simulink model "Reverse_Osmosis_2_pass_R2016a"  (R2022b)
settings: Solver=VariableStepAuto  StartTime=0.0  StopTime=7*3600  RelTol=1e-3
model workspace (MAT data in the model file):
  H2_D = 74
  H2_R = 4124.48151676
  H2_T = [-56.55 -50 -40 -30 -20 -10 -5 -4 -3 -2 -1 0 1 2 3 4 5 10 20 30 40 50 60 70 80 90 100 110 120 130 140 150 160 170 180 190 200 210 220 230 240 250 260 270 280 290 300 310 320 330 340 350]
  H2_h = [2783.66044046 2873.94181646 3012.62601981 3152.22537302 3292.62486344 3433.7213836 3504.50184296 3518.67512521 3532.85394544 3547.03822323 3561.22787913 3575.42283463 3589.62301216 3603.82833507 3618.03872764 3632.25411507 3646.47442344 3717.6472553 3860.32198735 4003.38288163 4146.77354613 4290.44463594 4434.35318484 4578.46197843 4722.73896833 4867.15672726 5011.69194457 5156.32496144 5301.03934494 5445.82149962 5590.66031514 5735.54684833 5880.47403768 6025.43644827 6170.43004499 6315.451992 6460.50047605 6605.57455183 6750.67400705 6895.79924544 7040.95118569 7186.13117474 7331.34091359 7476.58239436 7621.85784699 7767.16969457 7912.52051596 8057.91301484 8203.34999414 8348.83433523 8494.36898091 8639.95692183]
  H2_k = [142.834673487 146.602208511 152.236222043 157.732550942 163.09765294 168.338595937 170.914793442 171.426608923 171.937300227 172.446874689 172.955339635 173.462702375 173.968970204 174.474150403 174.978250232 175.481276935 175.983237736 178.477304495 183.389581256 188.206454189 192.934525091 197.580042888 202.148890501 206.646585109 211.078287131 215.448814629 219.762660868 224.024013436 228.236773895 232.404577248 236.530810786 240.618632037 244.670985681 248.690619345 252.680098287 256.641818973 260.578021603 264.490801638 268.382120403 272.253814814 276.107606319 279.945109096 283.767837587 287.577213413 291.374571729 295.161167068 298.938178719 302.706715675 306.467821201 310.222477041 313.971607306 317.716082068]
  H2_mu = [7.13280985169 7.28192581803 7.50683010986 7.72860158312 7.94743907375 8.16352107178 8.27057966039 8.29191522386 8.31322574339 8.33451136221 8.35577222214 8.37700846366 8.39822022586 8.41940764654 8.44057086215 8.46171000786 8.48282521754 8.58804682376 8.79676834159 9.00329345223 9.20773222364 9.41018554309 9.61074613692 9.80949945112 10.0065244149 10.2018941058 10.3956763308 10.5879341365 10.7787262582 10.9681075163 11.1561291684 11.3428392212 11.5282827091 11.7125019432 11.8955367341 12.0774245926 12.2582009096 12.4378991192 12.6165508457 12.7941860372 12.9708330866 13.1465189421 13.3212692073 13.4951082332 13.668059202 13.8401442043 14.0113843094 14.1817996299 14.3514093822 14.5202319407 14.6882848893 14.8555850676]
  N2_R = 296.802103844
  N2_T = [-56.55 -50 -40 -30 -20 -10 -5 -4 -3 -2 -1 0 1 2 3 4 5 10 20 30 40 50 60 70 80 90 100 110 120 130 140 150 160 170 180 190 200 210 220 230 240 250 260 270 280 290 300 310 320 330 340 350]
  N2_h = [224.312019476 231.141016529 241.564116975 251.984329606 262.402210767 272.818266127 278.025759131 279.06722248 280.10867517 281.150117667 282.191550441 283.232973957 284.274388686 285.315795097 286.357193658 287.39858484 288.439969116 293.646803475 304.060229226 314.473742204 324.887858161 335.303123494 345.720119003 356.139461811 366.561805672 376.987839946 387.41828743 397.853901301 408.295461341 418.743769659 429.199646055 439.663923199 450.137441735 460.621045431 471.115576471 481.621870952 492.140754651 502.673039103 513.219518026 523.780964099 534.358126107 544.951726469 555.562459109 566.190987693 576.837944198 587.503927793 598.18950402 608.895204248 619.621525378 630.368929765 641.137845362 651.928666026]
  N2_k = [19.6296532607 20.1533289725 20.9436243616 21.7231523445 22.4923063139 23.2514823267 23.6274403303 23.7023472872 23.7771601873 23.8518793809 23.9265052168 24.0010380424 24.0754782033 24.1498260439 24.2240819071 24.298246134 24.3723190645 24.7413260601 25.4726839899 26.1954347636 26.9098870601 27.616335804 28.3150627088 29.0063368423 29.6904152006 30.3675432786 31.0379556302 31.7018764132 32.3595199136 33.0110910506 33.656785857 34.2967919383 34.9312889073 35.560448797 36.1844364511 36.8034098926 37.4175206728 38.0269141997 38.6317300489 39.2321022558 39.8281595918 40.4200258249 41.0078199644 41.591656493 42.1716455849 42.7478933118 43.3205018374 43.8895696009 44.4551914905 45.0174590069 45.5764604183 46.1322809066]
  N2_mu = [13.7948920665 14.1367187352 14.6513506072 15.1575394446 15.6556177861 16.1459023391 16.3882166949 16.4364580271 16.4846261831 16.532721447 16.5807441017 16.6286944287 16.6765727079 16.7243792177 16.7721142355 16.8197780369 16.8673708962 17.1042805671 17.572933093 18.0349108462 18.4904598525 18.9398140034 19.38319572 19.820816593 20.2528779961 20.6795716689 21.1010802692 21.5175778944 21.9292305719 22.3361967211 22.7386275856 23.1366676392 23.5304549666 23.9201216192 24.3057939489 24.6875929203 25.0656344035 25.4400294479 25.8108845388 26.1783018382 26.5423794103 26.9032114332 27.260888397 27.615497291 27.9671217779 28.3158423592 28.6617365294 29.0048789219 29.3453414462 29.6831934166 30.0185016744 30.3513307024]
  O2_D = 18
  O2_R = 259.836612623
  O2_T = [-56.55 -50 -40 -30 -20 -10 -5 -4 -3 -2 -1 0 1 2 3 4 5 10 20 30 40 50 60 70 80 90 100 110 120 130 140 150 160 170 180 190 200 210 220 230 240 250 260 270 280 290 300 310 320 330 340 350]
  O2_h = [196.314045635 202.302438243 211.445560194 220.590899229 229.740231593 238.895348953 243.475641264 244.39194743 245.308340402 246.224821996 247.14139403 248.05805832 248.974816681 249.891670932 250.808622886 251.725674358 252.642827164 257.230174605 266.413508633 275.609852765 284.820965751 294.048557918 303.294277513 312.559698674 321.846311316 331.155513044 340.488603076 349.846778084 359.231129801 368.642644209 378.082202098 387.550580811 397.04845695 406.576409877 416.134925825 425.724402468 435.345153816 444.997415319 454.681349062 464.397049 474.144546127 483.92381355 493.734771414 503.577291639 513.451202454 523.356292707 533.292315938 543.258994208 553.256021689 563.283068012 573.339781379 583.425791441]
  O2_k = [19.6661951881 20.2224765128 21.0645207725 21.898029696 22.7232456338 23.5404090718 23.9460452976 24.0269406553 24.1077592592 24.1885013406 24.2691671302 24.349756858 24.4302707537 24.5107090462 24.5910719638 24.6713597344 24.751572585 25.1515209479 25.9459275198 26.7331962712 27.5135401678 28.2871691203 29.0542797087 29.8150645641 30.569709483 31.3183935589 32.0612893462 32.7985630479 33.5303747184 34.2568784759 34.9782227188 35.6945503443 36.4059989645 37.1127011203 37.81478449 38.5123720922 39.2055824827 39.8945299436 40.5793246667 41.2600729279 41.9368772562 42.6098365938 43.2790464498 43.9445990477 44.6065834647 45.2650857659 45.9201891311 46.5719739769 47.2205180715 47.8658966458 48.5081824976 49.1474460917]
  O2_mu = [15.7665575307 16.1727626079 16.7849249434 17.3877315055 17.9815180942 18.5666055809 18.8559834763 18.9136105725 18.9711555252 19.0286186248 19.0860001607 19.1433004205 19.2005196907 19.2576582565 19.3147164018 19.3716944089 19.4285925592 19.7118952085 20.2726692662 20.8258892364 21.3718096795 21.9106736607 22.4427133237 22.9681504449 23.4871969667 24.0000555078 24.5069198497 25.0079753989 25.5033996256 25.9933624783 26.4780267762 26.9575485797 27.4320775393 27.9017572254 28.3667254388 28.8271145028 29.2830515394 29.7346587283 30.1820535522 30.625349027 31.0646539191 31.5000729504 31.9317069915 32.3596532436 32.7840054112 33.2048538637 33.6222857893 34.0363853397 34.4472337669 34.8549095533 35.2594885333 35.6610440103]
  Op_Pressure = 40
  PEM_Efficiency = 0.9
  Power_suppy = 62000
  Sig = Simulink.Signal
  Sig.DataType = 'auto'
  Sig.Dimensions = -1
  Sig.DimensionsMode = 'auto'
  Sig.Complexity = 'auto'
  Sig.SampleTime = -1
  Sig.SamplingMode = 'auto'
  env_T = 15
  env_p = 0.101325
  exchanger_H = 2
  exchanger_L = 10
  exchanger_N_fins = 12000
  exchanger_N_tubes = 50
  exchanger_W = 0.5
  exchanger_air_area_fins = 11.5625
  exchanger_air_area_primary = 1.223125
  exchanger_eta_fin = 0.7
  exchanger_fin_spacing = 0.002
  exchanger_gap_H = 0.0192708333333
  exchanger_tube_H = 0.0015
  exchanger_tube_Leq = 2.5
  gas_pipe_D = 0.25
  solar_profile_power = [0; 0; 0; 0; 0; 0; 0.572; 13.1; 44.9; 74.5; 96.4; 100; 97.5; 89.5; 65.8; 34; 7.61; 0; 0; 0; 0; 0; 0; 0]
  solar_profile_time = [0; 3600; 7200; 10800; 14400; 18000; 21600; 25200; 28800; 32400; 36000; 39600; 43200; 46800; 50400; 54000; 57600; 61200; 64800; 68400; 72000; 75600; 79200; 82800]
  stack_D_gdl_A = 0.07
  stack_D_gdl_C = 0.07
  stack_alpha = 0.7
  stack_area = 175500
  stack_io = 1.3251
  stack_mea_cp = 870
  stack_mea_rho = 1800
  stack_membrane_MW = 1.1
  stack_membrane_rho = 2000
  stack_num_cells = 12500
  stack_num_channels = 8
  stack_t_gdl_A = 25
  stack_t_gdl_C = 250
  stack_t_membrane = 125
  stack_w_channels = 1
  water_pipe_D = 0.25
settings Model: Creator=mekala.suresh  LastModifiedBy=andres.lucht
settings SolverCC: MaxConsecutiveMinStep=2

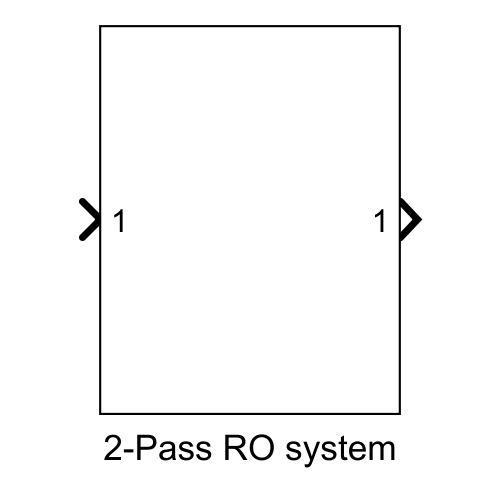
[thumbnail: Simulink's stored preview of the top-level diagram]
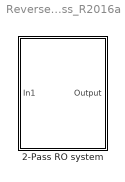
== system Reverse_Osmosis_2_pass_R2016a ==
  2-Pass RO system : Subsystem

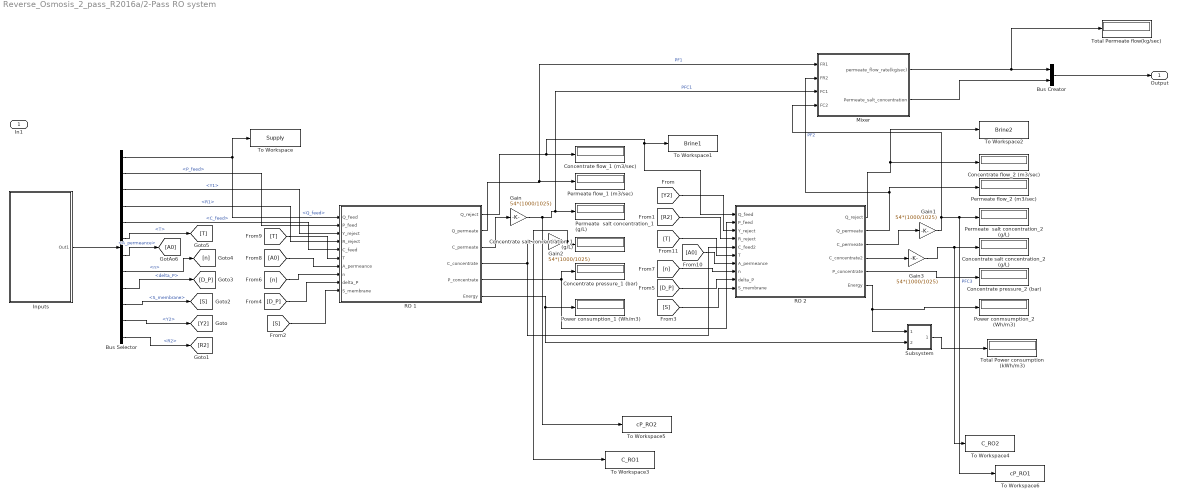
== system Reverse_Osmosis_2_pass_R2016a/2-Pass RO system ==
  In1 : Inport
  Bus Creator : BusCreator  Inputs=2
  Bus Selector : BusSelector  OutputSignals=Q_feed,P_feed,Y1,R1,C_feed,T,A_permeance,n,delta_P,S_membrane,Y2,R2
  Concentrate flow_1 (m3/sec) : Display
  Concentrate flow_2 (m3/sec) : Display
  Concentrate pressure_1 (bar) : Display
  Concentrate pressure_2 (bar) : Display
  Concentrate salt concentration_1 (g/L) : Display
  Concentrate salt concentration_2 (g/L) : Display
  Gain{,1..3} (4 alike) : Gain  Gain=54*(1000/1025)
  Inputs : Subsystem  mask{Q_feed=0.03, C_feed=40, T=27.85, P_feed=15.9, n=500, A_permeance=5.5e-13, S_membrane=35, Y1_reject=0.71, Y2_reject=0.50, R1_reject=0.98, R2_reject=0.99, delta_P=5}
      mask prompts: Q_feed "Flow rate(m3/sec)"; C_feed "Feed Salinity(mol/l)"; T "Water Temepreature(C°)"; P_feed "Feed Pressure(bar)"; n "Number of membrane modules"; A_permeance "Solvent permiability at 20°C en L/h/m2/bar"; S_membrane "Area of Membrane section (m2)"; Y1_reject "Conversion Rate RO1"; Y2_reject "Conversion Rate RO2"; R1_reject "Salt Rejection Rate RO1"; R2_reject "Salt Rejection Rate RO2"; delta_P "Pressure Drop(bar)"
      mask DialogControl DescGroupVar Prompt: Inputs
      mask DialogControl DescTextVar Prompt: Input parameters of RO systems for both the modules. Can edit the mask(UI) and the input parameters if more number of modules used in the RO system.(More detailed description about the model is available in the refered litarature and notes mentioned in Obsidian (Folder:Suresh Meklala >RO modeling))
      mask DialogControl ParameterGroupVar Prompt: Feed parameters
      mask DialogControl Container5 Prompt: RO Module 1 and 2 Design Parameters
  Mixer : Subsystem
  Permeate  salt concentration_1 (g/L) : Display
  Permeate  salt concentration_2 (g/L) : Display
  Permeate flow_1 (m3/sec) : Display
  "Permeate flow_2 (m3/sec) " : Display
  Power conmsumption_2 (Wh/m3) : Display
  Power consumption_1 (Wh/m3) : Display
  RO 1 : MATLAB Function  TreatAsAtomicUnit=on
  RO 2 : MATLAB Function  TreatAsAtomicUnit=on
  Subsystem : Subsystem
  To Workspace : ToWorkspace  VariableName=Supply  SampleTime=-1
  To Workspace1 : ToWorkspace  VariableName=Brine1  SampleTime=-1
  To Workspace2 : ToWorkspace  VariableName=Brine2  SampleTime=-1
  To Workspace3 : ToWorkspace  VariableName=C_RO1  SampleTime=-1
  To Workspace4 : ToWorkspace  VariableName=C_RO2  SampleTime=-1
  To Workspace5 : ToWorkspace  VariableName=cP_RO2  SampleTime=-1
  To Workspace6 : ToWorkspace  VariableName=cP_RO1  SampleTime=-1
  Total Permeate flow(kg/sec) : Display
  Total Power consumption (kWh/m3) : Display
  Output : Outport
  wires:
  RO 2/1(Q_reject) -> To Workspace2/1, Concentrate flow_2 (m3/sec)/1
  RO 2/3(C_permeate) -> Gain1/1
  [Y2] -> RO 2/3(Y_reject)
  RO 1/6(Energy) -> Subsystem/2(In2), Power consumption_1 (Wh/m3)/1
  Gain1/1 -> Mixer/4(FC2), To Workspace6/1, Permeate  salt concentration_2 (g/L)/1  "PFC3"
  Gain2/1 -> To Workspace3/1, Concentrate salt concentration_1 (g/L)/1
  Bus Selector/10 -> [S]  "<S_membrane>"
  Mixer/1(permeate_flow_rate(kg/sec)) -> Total Permeate flow(kg/sec)/1, Bus Creator/1
  Bus Selector/1 -> RO 1/1(Q_feed), To Workspace/1  "<Q_feed>"
  RO 1/4(C_concentrate) -> Gain2/1, RO 2/5(C_feed2)
  Bus Selector/12 -> [R2]  "<R2>"
  Bus Creator/1 -> Output/1
  Bus Selector/11 -> [Y2]  "<Y2>"
  Bus Selector/2 -> RO 1/2(P_feed)  "<P_feed>"
  RO 1/2(Q_permeate) -> Mixer/1(FR1), Permeate flow_1 (m3/sec)/1  "PF1"
  RO 2/4(C_concentrate2) -> Gain3/1
  Gain/1 -> To Workspace5/1, Mixer/3(FC1), Permeate  salt concentration_1 (g/L)/1  "PFC1"
  Mixer/2(Permeate_salt_concentration) -> Bus Creator/2
  [R2] -> RO 2/4(R_reject)
  [n] -> RO 2/8(n)
  RO 2/6(Energy) -> Power conmsumption_2 (Wh/m3)/1, Subsystem/1(In1)
  [A0] -> RO 1/7(A_permeance)
  [D_P] -> RO 2/9(delta_P)
  Bus Selector/9 -> [D_P]  "<delta_P>"
  [A0] -> RO 2/7(A_permeance)
  Bus Selector/6 -> [T]  "<T>"
  [T] -> RO 1/6(T)
  Gain3/1 -> To Workspace4/1, Concentrate salt concentration_2 (g/L)/1
  RO 1/1(Q_reject) -> RO 2/1(Q_feed), To Workspace1/1, Concentrate flow_1 (m3/sec)/1
  RO 1/5(P_concentrate) -> Concentrate pressure_1 (bar)/1, RO 2/2(P_feed)
  Bus Selector/5 -> RO 1/5(C_feed)  "<C_feed>"
  Subsystem/1(Out1) -> Total Power consumption (kWh/m3)/1
  [S] -> RO 1/10(S_membrane)
  RO 2/5(P_concentrate) -> Concentrate pressure_2 (bar)/1
  Bus Selector/7 -> [A0]  "<A_permeance>"
  Bus Selector/8 -> [n]  "<n>"
  RO 1/3(C_permeate) -> Gain/1
  [T] -> RO 2/6(T)
  Bus Selector/4 -> RO 1/4(R_reject)  "<R1>"
  [S] -> RO 2/10(S_membrane)
  RO 2/2(Q_permeate) -> Mixer/2(FR2), "Permeate flow_2 (m3/sec) "/1  "PF2"
  Inputs/1(Out1) -> Bus Selector/1
  Bus Selector/3 -> RO 1/3(Y_reject)  "<Y1>"
  [n] -> RO 1/8(n)
  [D_P] -> RO 1/9(delta_P)

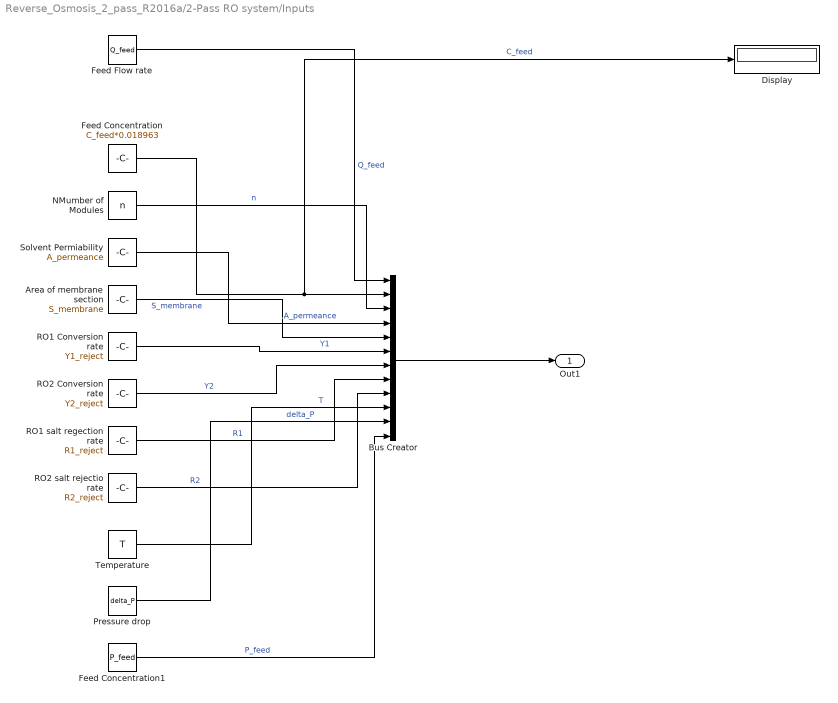
== system Reverse_Osmosis_2_pass_R2016a/2-Pass RO system/Inputs ==
  Area of membrane section : Constant  Value=S_membrane
  Bus Creator : BusCreator  Inputs=12
  Display : Display
  Feed Concentration : Constant  Value=C_feed*0.018963
  Feed Concentration1 : Constant  Value=P_feed
  Feed Flow rate : Constant  Value=Q_feed
  NMumber of Modules : Constant  Value=n
  Pressure drop : Constant  Value=delta_P
  RO1 Conversion rate : Constant  Value=Y1_reject
  RO1 salt regection rate : Constant  Value=R1_reject
  RO2 Conversion rate : Constant  Value=Y2_reject
  RO2 salt rejectio rate : Constant  Value=R2_reject
  Solvent Permiability : Constant  Value=A_permeance
  Temperature : Constant  Value=T
  Out1 : Outport
  wires:
  Feed Flow rate/1 -> Bus Creator/1  "Q_feed"
  Feed Concentration/1 -> Display/1, Bus Creator/2  "C_feed"
  NMumber of Modules/1 -> Bus Creator/3  "n"
  Solvent Permiability/1 -> Bus Creator/4  "A_permeance"
  Bus Creator/1 -> Out1/1
  Area of membrane section/1 -> Bus Creator/5  "S_membrane"
  RO1 Conversion rate/1 -> Bus Creator/6  "Y1"
  RO2 Conversion rate/1 -> Bus Creator/7  "Y2"
  RO1 salt regection rate/1 -> Bus Creator/8  "R1"
  RO2 salt rejectio rate/1 -> Bus Creator/9  "R2"
  Temperature/1 -> Bus Creator/10  "T"
  Pressure drop/1 -> Bus Creator/11  "delta_P"
  Feed Concentration1/1 -> Bus Creator/12  "P_feed"

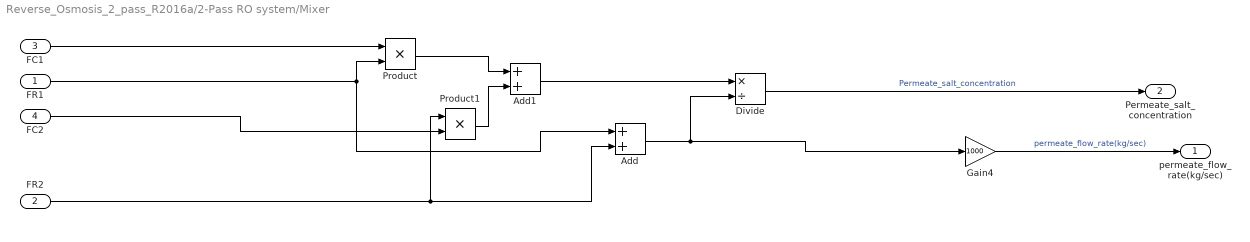
== system Reverse_Osmosis_2_pass_R2016a/2-Pass RO system/Mixer ==
  FR1 : Inport
  FR2 : Inport  Port=2
  FC1 : Inport  Port=3
  FC2 : Inport  Port=4
  Add : Sum
  Add1 : Sum
  Divide : Product  Inputs=*/
  Gain4 : Gain  Gain=1000
  Product : Product
  Product1 : Product
  permeate_flow_rate(kg/sec) : Outport
  Permeate_salt_concentration : Outport  Port=2
  wires:
  Add/1 -> Gain4/1, Divide/2
  Divide/1 -> Permeate_salt_concentration/1  "Permeate_salt_concentration"
  Product/1 -> Add1/1
  Product1/1 -> Add1/2
  Add1/1 -> Divide/1
  Gain4/1 -> permeate_flow_rate(kg/sec)/1  "permeate_flow_rate(kg/sec)"
  FC2/1 -> Product1/2
  FC1/1 -> Product/1
  FR1/1 -> Add/1, Product/2
  FR2/1 -> Add/2, Product1/1

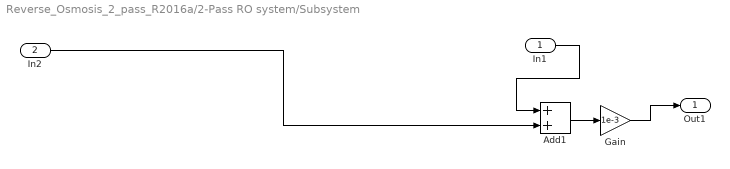
== system Reverse_Osmosis_2_pass_R2016a/2-Pass RO system/Subsystem ==
  In1 : Inport
  In2 : Inport  Port=2
  Add1 : Sum
  Gain : Gain  Gain=1e-3
  Out1 : Outport
  wires:
  Add1/1 -> Gain/1
  In1/1 -> Add1/1
  In2/1 -> Add1/2
  Gain/1 -> Out1/1

== matlab function Reverse_Osmosis_2_pass_R2016a/2-Pass RO system/RO 1 ==
  data: Q_feed input; Q_reject output; P_feed input; Y_reject input; R_reject input; C_feed input; Q_permeate output; C_permeate output; C_concentrate output; P_concentrate output; T input; A_permeance input; n input; delta_P input; Energy output; S_membrane input
function [Q_reject,Q_permeate,C_permeate,C_concentrate,P_concentrate,Energy]  = RO_module(Q_feed,P_feed,Y_reject,R_reject,C_feed,T,A_permeance,n,delta_P,S_membrane)

% all the equations are derived from the mass balance of the desalination
% process
Q_reject = Q_feed .* Y_reject;          % Concentrate flow rate
Q_permeate = Q_feed - Q_reject;         % Permiate flow rate
C_permeate = (1 - R_reject) .* C_feed;  % permiate concentration

% Calculate salt concentration in the concentrate stream using mass balance
C_concentrate = ((Q_feed .* C_feed) - (Q_permeate .* C_permeate)) ./ Q_reject; % Concentrate concentration
I= 2;                                   %number of ions dissociated in the case of an electrolyte

% Concentration of salts in mol/m3
R = 8.314;                                                                              % ideal gas constant J/mol.K

delta_phi_osmotic = I * R * T .* (C_concentrate - C_permeate);                          % osmotic pressure difference
A_water_permeance = A_permeance * exp(6.433 - 1885/T);                                  % m/s.Pa, water permeance constant
delta_P_p = ((delta_phi_osmotic) + (Q_permeate ./ (n*S_membrane*A_water_permeance)));   % bar, transmembrane pressure drop
P_permeate = 1 ; % P_feed - delta_P_transmembrane;                                      % bar, permeate pressure
%P_reject = P_feed-(n*delta_P_transmembrane);                                           % bar, concentrate pressure

P_concentrate = P_feed-delta_P ;

Energy = (((P_feed+P_concentrate)./2)*100)/(Y_reject.*0.8+3.6);

end

== matlab function Reverse_Osmosis_2_pass_R2016a/2-Pass RO system/RO 2 ==
  data: Q_feed input; Q_reject output; P_feed input; Y_reject input; R_reject input; C_feed2 input; Q_permeate output; C_permeate output; C_concentrate2 output; P_concentrate output; T input; A_permeance input; n input; delta_P input; Energy output; S_membrane input
function [Q_reject,Q_permeate,C_permeate,C_concentrate2,P_concentrate,Energy]  = RO_module(Q_feed,P_feed,Y_reject,R_reject,C_feed2,T,A_permeance,n,delta_P,S_membrane)

% all the equations are derived from the mass balance of the desalination
% process
Q_reject = Q_feed .* Y_reject;                                      % Concentrate flow rate
Q_permeate = Q_feed - Q_reject;                                     % Permiate flow rate
C_permeate = (1 - R_reject) .* C_feed2;                             % permiate concentration

% Calculate salt concentration in the concentrate stream using mass balance
C_concentrate2 = ((Q_feed .* C_feed2) - (Q_permeate .* C_permeate)) ./ Q_reject;        % Concentrate concentration
I= 2;    

%number of ions dissociated in the case of an electrolyte
% Concentration of salts in mol/m3
R = 8.314;                                                                              % ideal gas constant J/mol.K

delta_phi_osmotic = I * R * T * (C_concentrate2 - C_permeate);                          % osmotic pressure difference
A_water_permeance = A_permeance * exp(6.433 - 1885/T);                                  % m/s.Pa, water permeance constant
delta_P_p = ((delta_phi_osmotic) + (Q_permeate / (n*S_membrane*A_water_permeance)));    % bar, transmembrane pressure drop
P_permeate = 1 ; % P_feed - delta_P_transmembrane;                                      % bar, permeate pressure
%P_reject = P_feed-(n*delta_P_transmembrane);                                           % bar, concentrate pressure

P_concentrate = P_feed-delta_P ;

Energy = (((P_feed+P_concentrate)/2)*100)/(Y_reject*0.8+3.6);

end
